simulink model "eCS_Algo_Simulation_2015b_opti"  (R2015b)
settings: Solver=ode1  StartTime=0.0  StopTime=3  FixedStep=1/80000  RelTol=1e-3
PreLoadFcn:
  | if exist('tl_preloadfcn','file'), tl_preloadfcn(gcs,402); end
PostLoadFcn:
  | , if any(exist('dsrtsu_mdlpostloadfcn', 'file') == [2, 3, 6]), try dsrtsu_mdlpostloadfcn('Execute', bdroot); catch fprintf('Error in PostLoadFcn (dsrtsu_mdlpostloadfcn) for model "%s":\n %s\n', bdroot, lasterr); end, end,
  | if exist('tl_postloadfcn','file'), tl_postloadfcn(gcs,402); end
InitFcn:
  | Omegan=1.3024e+03;
  | xi=0.9; %0.48
  | K=0.1931;
  | K1=0.0198;
  | TauLocked=0.00255;
  | TauUnLocked=0.0042;
  | Kp=1/(2*K1);
  | Ki=Kp/((TauLocked+TauUnLocked)/2);
  | if exist('tlds_init','file'), tlds_init(gcs); end
StartFcn:
  | if exist('tlds_start','file'), tlds_start(gcs); end
StopFcn:
  | if exist('tlds_stop','file'), tlds_stop(gcs); end
model workspace (MAT data in the model file):
  au8PrevExecProfile = [0 0 0 0 0 0]
values from neighbouring files (symbols this model uses):
  AccSensor = 5    [Parameter_eCS_Algo.m]
  AlgoType = 0    [Parameter_eCS_Algo.m]
  Cxy = 1*0.017    (= 0.017)    [Acc_Init_SelV1.m]
  Cxz = 1*0.017    (= 0.017)    [Acc_Init_SelV1.m]
  Cyx = 1*0.017    (= 0.017)    [Acc_Init_SelV1.m]
  Cyz = 1*0.017    (= 0.017)    [Acc_Init_SelV1.m]
  Czx = 1*0.017    (= 0.017)    [Acc_Init_SelV1.m]
  Czy = 1*0.017    (= 0.017)    [Acc_Init_SelV1.m]
  Forced_Oscillation = 0    [Parameter_eCS_Algo.m]    (also in run_Rotation_sim.m = run)
  FreqTemperature = 10    [Acc_Init_SelV1.m]
  MaxSensorOffset = 0.3    [Acc_Init_SelV1.m]
  Mean_x_noise = 4e-3    (= 0.004)    [Acc_Init_SelV1.m]
  Mean_y_noise = 4e-3    (= 0.004)    [Acc_Init_SelV1.m]
  Mean_z_noise = 4e-3    (= 0.004)    [Acc_Init_SelV1.m]
  ODR = 8000    [Acc_Init_SelV1.m]
  offsetcorrection_on_off = 0    [Parameter_eCS_Algo.m]
  phi_pulse_rotation = 0    [Parameter_eCS_Algo.m]    (also in run_Rotation_sim.m = angle)
  pulsetype = 2    [Parameter_eCS_Algo.m]    (also in run_simulation.m = j; run_simulation_ActiveX.m = j)
  Range = 4    [Acc_Init_SelV1.m]
  sensitivity_optimisation = 0    [Parameter_eCS_Algo.m]
  TempBias = 0    [Acc_Init_SelV1.m]
  TemperatureAmp = 0    [Acc_Init_SelV1.m]
  Var_x_noise = 1.84e-9    (= 1.84e-09)    [Acc_Init_SelV1.m]
  Var_y_noise = 2.025e-09    [Acc_Init_SelV1.m]
  Var_z_noise = 1.374e-09    [Acc_Init_SelV1.m]
  w_x = 2*pi*F_x    (= 376.991118431)    [Acc_Init_SelV1.m]
  w_y = 2*pi*F_y    (= 376.991118431)    [Acc_Init_SelV1.m]
  w_z = 2*pi*F_z    (= 376.991118431)    [Acc_Init_SelV1.m]
  x_max_temp_drift = 0.061    [Acc_Init_SelV1.m]
  x_offset_enable = 0    [Acc_Init_SelV1.m]
  x_run_to_run_drift = 0.0    (= 0)    [Acc_Init_SelV1.m]
  x_temp_co_drift = 0.000    (= 0)    [Acc_Init_SelV1.m]
  Xi_x = 0.7    [Acc_Init_SelV1.m]
  Xi_y = 0.7    [Acc_Init_SelV1.m]
  Xi_z = 0.7    [Acc_Init_SelV1.m]
  y_max_temp_drift = 0.061    [Acc_Init_SelV1.m]
  y_offset_enable = 0    [Acc_Init_SelV1.m]
  y_run_to_run_drift = 0.0    (= 0)    [Acc_Init_SelV1.m]
  y_temp_co_drift = 0.000    (= 0)    [Acc_Init_SelV1.m]
  z_max_temp_drift = 0.13    [Acc_Init_SelV1.m]
  z_offset_enable = 0    [Acc_Init_SelV1.m]
  z_run_to_run_drift = 0.0    (= 0)    [Acc_Init_SelV1.m]
  z_temp_co_drift = 0.000    (= 0)    [Acc_Init_SelV1.m]
undefined symbols (not defined in the file or in its folder): ddv, DiscIntNeverNeededParam, gmw_roada_x__m_s__, gmw_roada_y__m_s__, gmw_roadtime_2kHz, KSF_50_a_x, KSF_50_a_y, KSF_50_time, KSG_30_a_x, KSG_30_a_y, KSG_30_time, Meldorf_HindenburgstraAcceleration_x__m_s_2_, Meldorf_HindenburgstraAcceleration_y__m_s_2_, Meldorf_HindenburgstraAcceleration_z__m_s_2_, Meldorf_HindenburgstraTime__s_, pulse_FF27, pulse_MPDB, pulse_ODB40, pulse_ODB64, pulse_USNCAP, pulsetime_FF27, pulsetime_MPDB, pulsetime_ODB40, pulsetime_ODB64, pulsetime_USNCAP, Rauasphalt_60_a_x, Rauasphalt_60_a_y, Rauasphalt_60_time, sigbuilder_block, VW_416_2kHza_x_2kHz, VW_416_2kHza_y_2kHz, VW_416_2kHztime_2kHz
libraries: simulink x20, tllib x14, tl_autosar_lib x9, simulink_extras x7, LIB_TF_G_12_StepControl x2, LIB_TF_G_111 x1, LIB_TF_G_112 x1
(part 5 of 8)

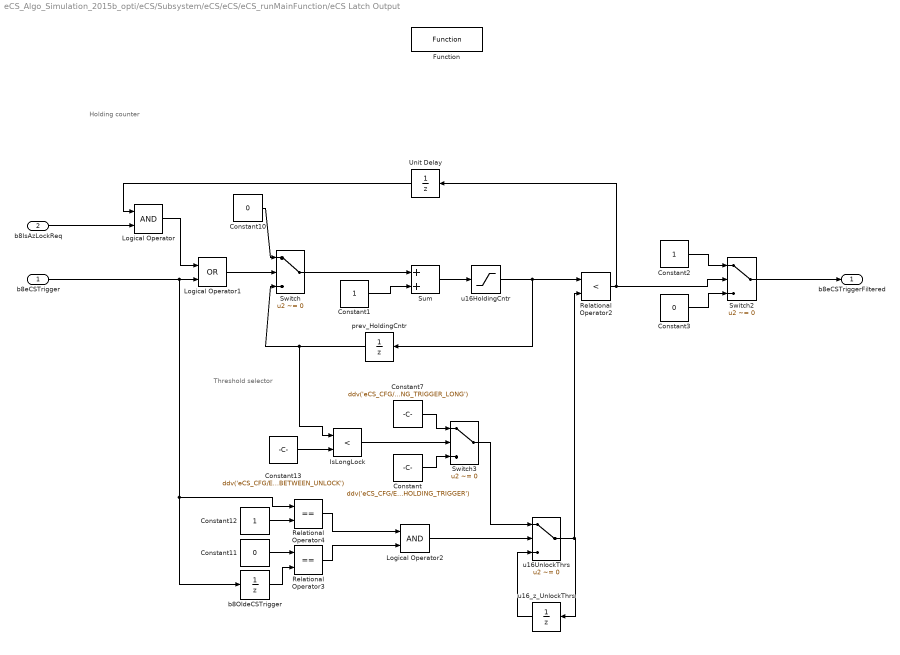
== system eCS_Algo_Simulation_2015b_opti/eCS/Subsystem/eCS/eCS/eCS_runMainFunction/eCS Latch Output ==
  note: Threshold selector
  note: Holding counter
  b8eCSTrigger : Inport
  b8IsAzLockReq : Inport  Port=2
  Constant : Constant  Value=ddv('eCS_CFG/ECS_HOLDING_TRIGGER')  mask(TL_Constant){data={'output',{'variable','eCS_CFG/ECS_HOLDING_TRIGGER'},'date',738573.71920614585}}
      settings: CopyFcn=if exist('tl_reset_reviewflag') == 2, tl_reset_reviewflag(gcbh); end  DeleteFcn=if exist('delete_tlblock','file')==2,delete_tlblock(gcbh);end  NameChangeFcn=if exist('rename_tlblock','file')==2,rename_tlblock(gcbh);end  OpenFcn=if exist('tl_open_blockdlg','file')==2,tl_open_blockdlg(gcbh);else,open_system(gcbh,'parameter');end
      mask Help: eval(['if exist(''tl_online_help'',''file'') == 2, tl_online_help(''Topic'',''TL_Constant''),else, web([''jar:file:///'',matlabroot,''/help/toolbox/simulink/help.jar!/slref/' lower(get_param(gcbh,'Blocktype')) '.html''], ''-helpbrowser''),end'])
      mask Display: plot([-0.1, 1.05, NaN, -0.1, 1.05],[.01, .01, NaN, .99, .99]);
  Constant1 : Constant  mask(TL_Constant){data={'date',738573.71920634259}}
      settings: CopyFcn=if exist('tl_reset_reviewflag') == 2, tl_reset_reviewflag(gcbh); end  DeleteFcn=if exist('delete_tlblock','file')==2,delete_tlblock(gcbh);end  NameChangeFcn=if exist('rename_tlblock','file')==2,rename_tlblock(gcbh);end  OpenFcn=if exist('tl_open_blockdlg','file')==2,tl_open_blockdlg(gcbh);else,open_system(gcbh,'parameter');end
      mask Help: eval(['if exist(''tl_online_help'',''file'') == 2, tl_online_help(''Topic'',''TL_Constant''),else, web([''jar:file:///'',matlabroot,''/help/toolbox/simulink/help.jar!/slref/' lower(get_param(gcbh,'Blocktype')) '.html''], ''-helpbrowser''),end'])
      mask Display: plot([-0.1, 1.05, NaN, -0.1, 1.05],[.01, .01, NaN, .99, .99]);
  Constant10 : Constant  Value=0  mask(TL_Constant){data={'date',738573.71920648147}}
      settings: CopyFcn=if exist('tl_reset_reviewflag') == 2, tl_reset_reviewflag(gcbh); end  DeleteFcn=if exist('delete_tlblock','file')==2,delete_tlblock(gcbh);end  NameChangeFcn=if exist('rename_tlblock','file')==2,rename_tlblock(gcbh);end  OpenFcn=if exist('tl_open_blockdlg','file')==2,tl_open_blockdlg(gcbh);else,open_system(gcbh,'parameter');end
      mask Help: eval(['if exist(''tl_online_help'',''file'') == 2, tl_online_help(''Topic'',''TL_Constant''),else, web([''jar:file:///'',matlabroot,''/help/toolbox/simulink/help.jar!/slref/' lower(get_param(gcbh,'Blocktype')) '.html''], ''-helpbrowser''),end'])
      mask Display: plot([-0.1, 1.05, NaN, -0.1, 1.05],[.01, .01, NaN, .99, .99]);
  Constant11 : Constant  Value=0  mask(TL_Constant){data={'date',738573.71920659719}}
      settings: CopyFcn=if exist('tl_reset_reviewflag') == 2, tl_reset_reviewflag(gcbh); end  DeleteFcn=if exist('delete_tlblock','file')==2,delete_tlblock(gcbh);end  NameChangeFcn=if exist('rename_tlblock','file')==2,rename_tlblock(gcbh);end  OpenFcn=if exist('tl_open_blockdlg','file')==2,tl_open_blockdlg(gcbh);else,open_system(gcbh,'parameter');end
      mask Help: eval(['if exist(''tl_online_help'',''file'') == 2, tl_online_help(''Topic'',''TL_Constant''),else, web([''jar:file:///'',matlabroot,''/help/toolbox/simulink/help.jar!/slref/' lower(get_param(gcbh,'Blocktype')) '.html''], ''-helpbrowser''),end'])
      mask Display: plot([-0.1, 1.05, NaN, -0.1, 1.05],[.01, .01, NaN, .99, .99]);
  Constant12 : Constant  mask(TL_Constant){data={'date',738573.71920671291}}
      settings: CopyFcn=if exist('tl_reset_reviewflag') == 2, tl_reset_reviewflag(gcbh); end  DeleteFcn=if exist('delete_tlblock','file')==2,delete_tlblock(gcbh);end  NameChangeFcn=if exist('rename_tlblock','file')==2,rename_tlblock(gcbh);end  OpenFcn=if exist('tl_open_blockdlg','file')==2,tl_open_blockdlg(gcbh);else,open_system(gcbh,'parameter');end
      mask Help: eval(['if exist(''tl_online_help'',''file'') == 2, tl_online_help(''Topic'',''TL_Constant''),else, web([''jar:file:///'',matlabroot,''/help/toolbox/simulink/help.jar!/slref/' lower(get_param(gcbh,'Blocktype')) '.html''], ''-helpbrowser''),end'])
      mask Display: plot([-0.1, 1.05, NaN, -0.1, 1.05],[.01, .01, NaN, .99, .99]);
  Constant13 : Constant  Value=ddv('eCS_CFG/ECS_DELAY_BETWEEN_UNLOCK')  mask(TL_Constant){data={'output',{'variable','eCS_CFG/ECS_DELAY_BETWEEN_UNLOCK'},'date',738573.71920692129}}
      settings: CopyFcn=if exist('tl_reset_reviewflag') == 2, tl_reset_reviewflag(gcbh); end  DeleteFcn=if exist('delete_tlblock','file')==2,delete_tlblock(gcbh);end  NameChangeFcn=if exist('rename_tlblock','file')==2,rename_tlblock(gcbh);end  OpenFcn=if exist('tl_open_blockdlg','file')==2,tl_open_blockdlg(gcbh);else,open_system(gcbh,'parameter');end
      mask Help: eval(['if exist(''tl_online_help'',''file'') == 2, tl_online_help(''Topic'',''TL_Constant''),else, web([''jar:file:///'',matlabroot,''/help/toolbox/simulink/help.jar!/slref/' lower(get_param(gcbh,'Blocktype')) '.html''], ''-helpbrowser''),end'])
      mask Display: plot([-0.1, 1.05, NaN, -0.1, 1.05],[.01, .01, NaN, .99, .99]);
  Constant2 : Constant  mask(TL_Constant){data={'date',738573.71920706017}}
      settings: CopyFcn=if exist('tl_reset_reviewflag') == 2, tl_reset_reviewflag(gcbh); end  DeleteFcn=if exist('delete_tlblock','file')==2,delete_tlblock(gcbh);end  NameChangeFcn=if exist('rename_tlblock','file')==2,rename_tlblock(gcbh);end  OpenFcn=if exist('tl_open_blockdlg','file')==2,tl_open_blockdlg(gcbh);else,open_system(gcbh,'parameter');end
      mask Help: eval(['if exist(''tl_online_help'',''file'') == 2, tl_online_help(''Topic'',''TL_Constant''),else, web([''jar:file:///'',matlabroot,''/help/toolbox/simulink/help.jar!/slref/' lower(get_param(gcbh,'Blocktype')) '.html''], ''-helpbrowser''),end'])
      mask Display: plot([-0.1, 1.05, NaN, -0.1, 1.05],[.01, .01, NaN, .99, .99]);
  Constant3 : Constant  Value=0  mask(TL_Constant){data={'date',738573.71920717589}}
      settings: CopyFcn=if exist('tl_reset_reviewflag') == 2, tl_reset_reviewflag(gcbh); end  DeleteFcn=if exist('delete_tlblock','file')==2,delete_tlblock(gcbh);end  NameChangeFcn=if exist('rename_tlblock','file')==2,rename_tlblock(gcbh);end  OpenFcn=if exist('tl_open_blockdlg','file')==2,tl_open_blockdlg(gcbh);else,open_system(gcbh,'parameter');end
      mask Help: eval(['if exist(''tl_online_help'',''file'') == 2, tl_online_help(''Topic'',''TL_Constant''),else, web([''jar:file:///'',matlabroot,''/help/toolbox/simulink/help.jar!/slref/' lower(get_param(gcbh,'Blocktype')) '.html''], ''-helpbrowser''),end'])
      mask Display: plot([-0.1, 1.05, NaN, -0.1, 1.05],[.01, .01, NaN, .99, .99]);
  Constant7 : Constant  Value=ddv('eCS_CFG/ECS_HOLDING_TRIGGER_LONG')  mask(TL_Constant){data={'output',{'variable','eCS_CFG/ECS_HOLDING_TRIGGER_LONG'},'date',738573.71920729172}}
      settings: CopyFcn=if exist('tl_reset_reviewflag') == 2, tl_reset_reviewflag(gcbh); end  DeleteFcn=if exist('delete_tlblock','file')==2,delete_tlblock(gcbh);end  NameChangeFcn=if exist('rename_tlblock','file')==2,rename_tlblock(gcbh);end  OpenFcn=if exist('tl_open_blockdlg','file')==2,tl_open_blockdlg(gcbh);else,open_system(gcbh,'parameter');end
      mask Help: eval(['if exist(''tl_online_help'',''file'') == 2, tl_online_help(''Topic'',''TL_Constant''),else, web([''jar:file:///'',matlabroot,''/help/toolbox/simulink/help.jar!/slref/' lower(get_param(gcbh,'Blocktype')) '.html''], ''-helpbrowser''),end'])
      mask Display: plot([-0.1, 1.05, NaN, -0.1, 1.05],[.01, .01, NaN, .99, .99]);
  Function : tllib/Function  data={'stepfunctionname','eCS_LatchTrigger','date',738077.45310667821}  displayString=FUNCTION
  IsLongLock : RelationalOperator  Operator=<  OutDataTypeStr=boolean  mask(TL_RelationalOperator){data={'date',738573.71920749999}}
      settings: DeleteFcn=if exist('delete_tlblock','file')==2,delete_tlblock(gcbh);end  NameChangeFcn=if exist('rename_tlblock','file')==2,rename_tlblock(gcbh);end  OpenFcn=if exist('tl_open_blockdlg','file')==2,tl_open_blockdlg(gcbh);else,open_system(gcbh,'parameter');end
      mask Help: eval(['if exist(''tl_online_help'',''file'') == 2, tl_online_help(''Topic'',''TL_RelationalOperator''),else, web([''jar:file:///'',matlabroot,''/help/toolbox/simulink/help.jar!/slref/' lower(get_param(gcbh,'Blocktype')) '.html''], ''-helpbrowser''),end'])
      mask Display: plot([-0.1, 1.05, NaN, -0.1, 1.05],[.01, .01, NaN, .99, .99]);
  Logical Operator : Logic  AllPortsSameDT=off  OutDataTypeStr=boolean  mask(TL_LogicalOperator){data={'date',738573.71920762735}}
      settings: DeleteFcn=if exist('delete_tlblock','file')==2,delete_tlblock(gcbh);end  NameChangeFcn=if exist('rename_tlblock','file')==2,rename_tlblock(gcbh);end  OpenFcn=if exist('tl_open_blockdlg','file')==2,tl_open_blockdlg(gcbh);else,open_system(gcbh,'parameter');end
      mask Help: eval(['if exist(''tl_online_help'',''file'') == 2, tl_online_help(''Topic'',''TL_LogicalOperator''),else, web([''jar:file:///'',matlabroot,''/help/toolbox/simulink/help.jar!/slref/' lower(get_param(gcbh,'Blocktype')) '.html''], ''-helpbrowser''),end'])
      mask Display: plot([-0.1, 1.05, NaN, -0.1, 1.05],[.01, .01, NaN, .99, .99]);
  Logical Operator1 : Logic  Operator=OR  AllPortsSameDT=off  OutDataTypeStr=boolean  mask(TL_LogicalOperator){data={'date',738573.71920774307}}
      settings: DeleteFcn=if exist('delete_tlblock','file')==2,delete_tlblock(gcbh);end  NameChangeFcn=if exist('rename_tlblock','file')==2,rename_tlblock(gcbh);end  OpenFcn=if exist('tl_open_blockdlg','file')==2,tl_open_blockdlg(gcbh);else,open_system(gcbh,'parameter');end
      mask Help: eval(['if exist(''tl_online_help'',''file'') == 2, tl_online_help(''Topic'',''TL_LogicalOperator''),else, web([''jar:file:///'',matlabroot,''/help/toolbox/simulink/help.jar!/slref/' lower(get_param(gcbh,'Blocktype')) '.html''], ''-helpbrowser''),end'])
      mask Display: plot([-0.1, 1.05, NaN, -0.1, 1.05],[.01, .01, NaN, .99, .99]);
  Logical Operator2 : Logic  AllPortsSameDT=off  OutDataTypeStr=boolean  mask(TL_LogicalOperator){data={'date',738573.71920785878}}
      settings: DeleteFcn=if exist('delete_tlblock','file')==2,delete_tlblock(gcbh);end  NameChangeFcn=if exist('rename_tlblock','file')==2,rename_tlblock(gcbh);end  OpenFcn=if exist('tl_open_blockdlg','file')==2,tl_open_blockdlg(gcbh);else,open_system(gcbh,'parameter');end
      mask Help: eval(['if exist(''tl_online_help'',''file'') == 2, tl_online_help(''Topic'',''TL_LogicalOperator''),else, web([''jar:file:///'',matlabroot,''/help/toolbox/simulink/help.jar!/slref/' lower(get_param(gcbh,'Blocktype')) '.html''], ''-helpbrowser''),end'])
      mask Display: plot([-0.1, 1.05, NaN, -0.1, 1.05],[.01, .01, NaN, .99, .99]);
  Relational Operator2 : RelationalOperator  Operator=<  OutDataTypeStr=boolean  mask(TL_RelationalOperator){data={'date',738573.71920802083}}
      settings: DeleteFcn=if exist('delete_tlblock','file')==2,delete_tlblock(gcbh);end  NameChangeFcn=if exist('rename_tlblock','file')==2,rename_tlblock(gcbh);end  OpenFcn=if exist('tl_open_blockdlg','file')==2,tl_open_blockdlg(gcbh);else,open_system(gcbh,'parameter');end
      mask Help: eval(['if exist(''tl_online_help'',''file'') == 2, tl_online_help(''Topic'',''TL_RelationalOperator''),else, web([''jar:file:///'',matlabroot,''/help/toolbox/simulink/help.jar!/slref/' lower(get_param(gcbh,'Blocktype')) '.html''], ''-helpbrowser''),end'])
      mask Display: plot([-0.1, 1.05, NaN, -0.1, 1.05],[.01, .01, NaN, .99, .99]);
  Relational Operator3 : RelationalOperator  Operator===  OutDataTypeStr=boolean  mask(TL_RelationalOperator){data={'date',738573.71920814819}}
      settings: DeleteFcn=if exist('delete_tlblock','file')==2,delete_tlblock(gcbh);end  NameChangeFcn=if exist('rename_tlblock','file')==2,rename_tlblock(gcbh);end  OpenFcn=if exist('tl_open_blockdlg','file')==2,tl_open_blockdlg(gcbh);else,open_system(gcbh,'parameter');end
      mask Help: eval(['if exist(''tl_online_help'',''file'') == 2, tl_online_help(''Topic'',''TL_RelationalOperator''),else, web([''jar:file:///'',matlabroot,''/help/toolbox/simulink/help.jar!/slref/' lower(get_param(gcbh,'Blocktype')) '.html''], ''-helpbrowser''),end'])
      mask Display: plot([-0.1, 1.05, NaN, -0.1, 1.05],[.01, .01, NaN, .99, .99]);
  Relational Operator4 : RelationalOperator  Operator===  OutDataTypeStr=boolean  mask(TL_RelationalOperator){data={'date',738573.71920833329}}
      settings: DeleteFcn=if exist('delete_tlblock','file')==2,delete_tlblock(gcbh);end  NameChangeFcn=if exist('rename_tlblock','file')==2,rename_tlblock(gcbh);end  OpenFcn=if exist('tl_open_blockdlg','file')==2,tl_open_blockdlg(gcbh);else,open_system(gcbh,'parameter');end
      mask Help: eval(['if exist(''tl_online_help'',''file'') == 2, tl_online_help(''Topic'',''TL_RelationalOperator''),else, web([''jar:file:///'',matlabroot,''/help/toolbox/simulink/help.jar!/slref/' lower(get_param(gcbh,'Blocktype')) '.html''], ''-helpbrowser''),end'])
      mask Display: plot([-0.1, 1.05, NaN, -0.1, 1.05],[.01, .01, NaN, .99, .99]);
  Sum : Sum  mask(TL_Sum){data={'output',{'type','UInt16'},'date',738573.71920846065}}
      settings: CopyFcn=if exist('tl_reset_reviewflag') == 2, tl_reset_reviewflag(gcbh); end  DeleteFcn=if exist('delete_tlblock','file')==2,delete_tlblock(gcbh);end  NameChangeFcn=if exist('rename_tlblock','file')==2,rename_tlblock(gcbh);end  OpenFcn=if exist('tl_open_blockdlg','file')==2,tl_open_blockdlg(gcbh);else,open_system(gcbh,'parameter');end
      mask Help: eval(['if exist(''tl_online_help'',''file'') == 2, tl_online_help(''Topic'',''TL_Sum''),else, web([''jar:file:///'',matlabroot,''/help/toolbox/simulink/help.jar!/slref/' lower(get_param(gcbh,'Blocktype')) '.html''], ''-helpbrowser''),end'])
      mask Display: plot([-0.1, 1.05, NaN, -0.1, 1.05],[.01, .01, NaN, .99, .99]);
  Switch : Switch  Criteria=u2 ~= 0  mask(TL_Switch){data={'output',{'type','UInt16'},'date',738573.71920854168}}
      settings: CopyFcn=if exist('tl_reset_reviewflag') == 2, tl_reset_reviewflag(gcbh); end  DeleteFcn=if exist('delete_tlblock','file')==2,delete_tlblock(gcbh);end  NameChangeFcn=if exist('rename_tlblock','file')==2,rename_tlblock(gcbh);end  OpenFcn=if exist('tl_open_blockdlg','file')==2,tl_open_blockdlg(gcbh);else,open_system(gcbh,'parameter');end
      mask Help: eval(['if exist(''tl_online_help'',''file'') == 2, tl_online_help(''Topic'',''TL_Switch''),else, web([''jar:file:///'',matlabroot,''/help/toolbox/simulink/help.jar!/slref/' lower(get_param(gcbh,'Blocktype')) '.html''], ''-helpbrowser''),end'])
      mask Display: plot([-0.1, 1.05, NaN, -0.1, 1.05],[.01, .01, NaN, .99, .99]);
  Switch2 : Switch  Criteria=u2 ~= 0  mask(TL_Switch){data={'output',{'type','Bool'},'date',738573.71920869208}}
      settings: CopyFcn=if exist('tl_reset_reviewflag') == 2, tl_reset_reviewflag(gcbh); end  DeleteFcn=if exist('delete_tlblock','file')==2,delete_tlblock(gcbh);end  NameChangeFcn=if exist('rename_tlblock','file')==2,rename_tlblock(gcbh);end  OpenFcn=if exist('tl_open_blockdlg','file')==2,tl_open_blockdlg(gcbh);else,open_system(gcbh,'parameter');end
      mask Help: eval(['if exist(''tl_online_help'',''file'') == 2, tl_online_help(''Topic'',''TL_Switch''),else, web([''jar:file:///'',matlabroot,''/help/toolbox/simulink/help.jar!/slref/' lower(get_param(gcbh,'Blocktype')) '.html''], ''-helpbrowser''),end'])
      mask Display: plot([-0.1, 1.05, NaN, -0.1, 1.05],[.01, .01, NaN, .99, .99]);
  Switch3 : Switch  Criteria=u2 ~= 0  mask(TL_Switch){data={'output',{'type','UInt16'},'date',738573.7192089468}}
      settings: CopyFcn=if exist('tl_reset_reviewflag') == 2, tl_reset_reviewflag(gcbh); end  DeleteFcn=if exist('delete_tlblock','file')==2,delete_tlblock(gcbh);end  NameChangeFcn=if exist('rename_tlblock','file')==2,rename_tlblock(gcbh);end  OpenFcn=if exist('tl_open_blockdlg','file')==2,tl_open_blockdlg(gcbh);else,open_system(gcbh,'parameter');end
      mask Help: eval(['if exist(''tl_online_help'',''file'') == 2, tl_online_help(''Topic'',''TL_Switch''),else, web([''jar:file:///'',matlabroot,''/help/toolbox/simulink/help.jar!/slref/' lower(get_param(gcbh,'Blocktype')) '.html''], ''-helpbrowser''),end'])
      mask Display: plot([-0.1, 1.05, NaN, -0.1, 1.05],[.01, .01, NaN, .99, .99]);
  Unit Delay : UnitDelay  SampleTime=-1  mask(TL_UnitDelay){data={'output',{'type','Bool'},'state',{'type','Bool'},'date',738573.71920909721}}
      settings: CopyFcn=if exist('tl_reset_reviewflag') == 2, tl_reset_reviewflag(gcbh); end  DeleteFcn=if exist('delete_tlblock','file')==2,delete_tlblock(gcbh);end  NameChangeFcn=if exist('rename_tlblock','file')==2,rename_tlblock(gcbh);end  OpenFcn=if exist('tl_open_blockdlg','file')==2,tl_open_blockdlg(gcbh);else,open_system(gcbh,'parameter');end
      mask Help: eval(['if exist(''tl_online_help'',''file'') == 2, tl_online_help(''Topic'',''TL_UnitDelay''),else, web([''jar:file:///'',matlabroot,''/help/toolbox/simulink/help.jar!/slref/' lower(get_param(gcbh,'Blocktype')) '.html''], ''-helpbrowser''),end'])
      mask Display: plot([-0.1, 1.05, NaN, -0.1, 1.05],[.01, .01, NaN, .99, .99]);
  b8OldeCSTrigger : UnitDelay  SampleTime=-1  mask(TL_UnitDelay){data={'date',738573.71920924773}}
      settings: CopyFcn=if exist('tl_reset_reviewflag') == 2, tl_reset_reviewflag(gcbh); end  DeleteFcn=if exist('delete_tlblock','file')==2,delete_tlblock(gcbh);end  NameChangeFcn=if exist('rename_tlblock','file')==2,rename_tlblock(gcbh);end  OpenFcn=if exist('tl_open_blockdlg','file')==2,tl_open_blockdlg(gcbh);else,open_system(gcbh,'parameter');end
      mask Help: eval(['if exist(''tl_online_help'',''file'') == 2, tl_online_help(''Topic'',''TL_UnitDelay''),else, web([''jar:file:///'',matlabroot,''/help/toolbox/simulink/help.jar!/slref/' lower(get_param(gcbh,'Blocktype')) '.html''], ''-helpbrowser''),end'])
      mask Display: plot([-0.1, 1.05, NaN, -0.1, 1.05],[.01, .01, NaN, .99, .99]);
  prev_HoldingCntr : UnitDelay  SampleTime=-1  mask(TL_UnitDelay){data={'output',{'type','UInt16'},'state',{'type','UInt16'},'date',738573.71920953703}}
      settings: CopyFcn=if exist('tl_reset_reviewflag') == 2, tl_reset_reviewflag(gcbh); end  DeleteFcn=if exist('delete_tlblock','file')==2,delete_tlblock(gcbh);end  NameChangeFcn=if exist('rename_tlblock','file')==2,rename_tlblock(gcbh);end  OpenFcn=if exist('tl_open_blockdlg','file')==2,tl_open_blockdlg(gcbh);else,open_system(gcbh,'parameter');end
      mask Help: eval(['if exist(''tl_online_help'',''file'') == 2, tl_online_help(''Topic'',''TL_UnitDelay''),else, web([''jar:file:///'',matlabroot,''/help/toolbox/simulink/help.jar!/slref/' lower(get_param(gcbh,'Blocktype')) '.html''], ''-helpbrowser''),end'])
      mask Display: plot([-0.1, 1.05, NaN, -0.1, 1.05],[.01, .01, NaN, .99, .99]);
  u16HoldingCntr : Saturate  UpperLimit=4000  LowerLimit=0  mask(TL_Saturate){data={'logdata',{'loggingmode',1},'output',{'type','UInt16'},'date',738573.71920969908}}
      settings: CopyFcn=if exist('tl_reset_reviewflag') == 2, tl_reset_reviewflag(gcbh); end  DeleteFcn=if exist('delete_tlblock','file')==2,delete_tlblock(gcbh);end  NameChangeFcn=if exist('rename_tlblock','file')==2,rename_tlblock(gcbh);end  OpenFcn=if exist('tl_open_blockdlg','file')==2,tl_open_blockdlg(gcbh);else,open_system(gcbh,'parameter');end
      mask Help: eval(['if exist(''tl_online_help'',''file'') == 2, tl_online_help(''Topic'',''TL_Saturate''),else, web([''jar:file:///'',matlabroot,''/help/toolbox/simulink/help.jar!/slref/' lower(get_param(gcbh,'Blocktype')) '.html''], ''-helpbrowser''),end'])
      mask Display: plot([-0.1, 1.05, NaN, -0.1, 1.05],[.01, .01, NaN, .99, .99]);
  u16UnlockThrs : Switch  Criteria=u2 ~= 0  mask(TL_Switch){data={'logdata',{'loggingmode',1},'output',{'type','UInt16'},'date',738573.71920981479}}
      settings: CopyFcn=if exist('tl_reset_reviewflag') == 2, tl_reset_reviewflag(gcbh); end  DeleteFcn=if exist('delete_tlblock','file')==2,delete_tlblock(gcbh);end  NameChangeFcn=if exist('rename_tlblock','file')==2,rename_tlblock(gcbh);end  OpenFcn=if exist('tl_open_blockdlg','file')==2,tl_open_blockdlg(gcbh);else,open_system(gcbh,'parameter');end
      mask Help: eval(['if exist(''tl_online_help'',''file'') == 2, tl_online_help(''Topic'',''TL_Switch''),else, web([''jar:file:///'',matlabroot,''/help/toolbox/simulink/help.jar!/slref/' lower(get_param(gcbh,'Blocktype')) '.html''], ''-helpbrowser''),end'])
      mask Display: plot([-0.1, 1.05, NaN, -0.1, 1.05],[.01, .01, NaN, .99, .99]);
  u16_z_UnlockThrs : UnitDelay  SampleTime=-1  mask(TL_UnitDelay){data={'output',{'type','UInt16'},'state',{'type','UInt16'},'date',738573.71921006939}}
      settings: CopyFcn=if exist('tl_reset_reviewflag') == 2, tl_reset_reviewflag(gcbh); end  DeleteFcn=if exist('delete_tlblock','file')==2,delete_tlblock(gcbh);end  NameChangeFcn=if exist('rename_tlblock','file')==2,rename_tlblock(gcbh);end  OpenFcn=if exist('tl_open_blockdlg','file')==2,tl_open_blockdlg(gcbh);else,open_system(gcbh,'parameter');end
      mask Help: eval(['if exist(''tl_online_help'',''file'') == 2, tl_online_help(''Topic'',''TL_UnitDelay''),else, web([''jar:file:///'',matlabroot,''/help/toolbox/simulink/help.jar!/slref/' lower(get_param(gcbh,'Blocktype')) '.html''], ''-helpbrowser''),end'])
      mask Display: plot([-0.1, 1.05, NaN, -0.1, 1.05],[.01, .01, NaN, .99, .99]);
  b8eCSTriggerFiltered : Outport
  wires:
  b8eCSTrigger/1 -> Relational Operator4/1, b8OldeCSTrigger/1, Logical Operator1/2
  Switch/1 -> Sum/1
  Constant1/1 -> Sum/2
  Sum/1 -> u16HoldingCntr/1
  u16HoldingCntr/1 -> Relational Operator2/1, prev_HoldingCntr/1
  prev_HoldingCntr/1 -> IsLongLock/1, Switch/3
  Constant7/1 -> Switch3/1
  Constant/1 -> Switch3/3
  Switch2/1 -> b8eCSTriggerFiltered/1
  Constant10/1 -> Switch/1
  Relational Operator4/1 -> Logical Operator2/1
  Relational Operator3/1 -> Logical Operator2/2
  Constant11/1 -> Relational Operator3/1
  b8OldeCSTrigger/1 -> Relational Operator3/2
  Constant12/1 -> Relational Operator4/2
  Logical Operator2/1 -> u16UnlockThrs/2
  Switch3/1 -> u16UnlockThrs/1
  Constant13/1 -> IsLongLock/2
  IsLongLock/1 -> Switch3/2
  u16UnlockThrs/1 -> Relational Operator2/2, u16_z_UnlockThrs/1
  u16_z_UnlockThrs/1 -> u16UnlockThrs/3
  Relational Operator2/1 -> Unit Delay/1, Switch2/2
  Constant2/1 -> Switch2/1
  Constant3/1 -> Switch2/3
  b8IsAzLockReq/1 -> Logical Operator/2
  Logical Operator1/1 -> Switch/2
  Logical Operator/1 -> Logical Operator1/1
  Unit Delay/1 -> Logical Operator/1

== system eCS_Algo_Simulation_2015b_opti/FSM/Subsystem/FSM/FSM/FSM_runCheckVehicleInputs/For Iterator Subsystem/FSM_runCheckModeStatus  ==
  u32ModesToCheck : Inport  PortDimensions=1  mask(TL_Inport){data={'output',{'variable','LOCAL_FSM/u32ModesToCheck'},'date',738799.46899457171}}
      settings: CopyFcn=if exist('tl_reset_reviewflag','file')==2,tl_reset_reviewflag(gcbh);end  DeleteFcn=if exist('delete_tlblock','file')==2,delete_tlblock(gcbh);end  NameChangeFcn=if exist('rename_tlblock','file')==2,rename_tlblock(gcbh);end  OpenFcn=if exist('tl_open_blockdlg','file')==2,tl_open_blockdlg(gcbh);else,open_system(gcbh,'parameter');end
      mask Help: eval(['if exist(''tl_online_help'',''file'') == 2, tl_online_help(''Topic'',''TL_Inport''),else, web([''jar:file:///'',matlabroot,''/help/toolbox/simulink/help.jar!/slref/' lower(get_param(gcbh,'Blocktype')) '.html''], ''-helpbrowser''),end'])
      mask Display: plot([0.2 0.35 NaN 0.65 0.8],[0 1 NaN 0 1]);
  Constant : Constant  Value=ddv('Common/B_TRUE')  mask(TL_Constant){data={'output',{'variable','Common/B_TRUE'},'date',738790.47864616895}}
      settings: CopyFcn=if exist('tl_reset_reviewflag','file')==2,tl_reset_reviewflag(gcbh);end  DeleteFcn=if exist('delete_tlblock','file')==2,delete_tlblock(gcbh);end  NameChangeFcn=if exist('rename_tlblock','file')==2,rename_tlblock(gcbh);end  OpenFcn=if exist('tl_open_blockdlg','file')==2,tl_open_blockdlg(gcbh);else,open_system(gcbh,'parameter');end
      mask Help: eval(['if exist(''tl_online_help'',''file'') == 2, tl_online_help(''Topic'',''TL_Constant''),else, web([''jar:file:///'',matlabroot,''/help/toolbox/simulink/help.jar!/slref/' lower(get_param(gcbh,'Blocktype')) '.html''], ''-helpbrowser''),end'])
      mask Display: plot([-0.1, 1.05, NaN, -0.1, 1.05],[.01, .01, NaN, .99, .99]);
  Function : tllib/Function  data={'stepfunctionname','FSM_runCheckModeStatus','stepfunctionclass','EXTERN_FCN','initfunctionname','INIT_FSM_runCheckModeStatus','functionarglist',{'u32ModesToCheck';'FSM_b8_ModeStatusResult'},'autosar',{'softwarecomponent','AUTOLIV/SoftwareComponents/FSM/FSM','runnable','FSM_runCheckModeStatus'},'date',738800.40523146989}  displayString=FUNCTION
  Terminator : Terminator
  FSM_b8_ModeStatusResult : Outport  PortDimensions=1  mask(TL_Outport){data={'output',{'variable','LOCAL_FSM/FSM_b8_ModeStatusResult'},'date',738798.55828084494}}
      settings: CopyFcn=if exist('tl_reset_reviewflag','file')==2,tl_reset_reviewflag(gcbh);end  DeleteFcn=if exist('delete_tlblock','file')==2,delete_tlblock(gcbh);end  NameChangeFcn=if exist('rename_tlblock','file')==2,rename_tlblock(gcbh);end  OpenFcn=if exist('tl_open_blockdlg','file')==2,tl_open_blockdlg(gcbh);else,open_system(gcbh,'parameter');end
      mask Help: eval(['if exist(''tl_online_help'',''file'') == 2, tl_online_help(''Topic'',''TL_Outport''),else, web([''jar:file:///'',matlabroot,''/help/toolbox/simulink/help.jar!/slref/' lower(get_param(gcbh,'Blocktype')) '.html''], ''-helpbrowser''),end'])
      mask Display: plot([0.2 0.35 NaN 0.65 0.8],[0 1 NaN 0 1]);
  wires:
  Constant/1 -> FSM_b8_ModeStatusResult/1
  u32ModesToCheck/1 -> Terminator/1

== system eCS_Algo_Simulation_2015b_opti/FSM/Subsystem/FSM/FSM/FSM_runMainFunction/ExecuteState/State Default ==
  Action Port : ActionPort  ActionType=default
  Constant1 : Constant  Value=ddv('FSM/Macros/KU8_PROFILE_NONE')  mask(TL_Constant){data={'output',{'variable','FSM/Macros/KU8_PROFILE_NONE'},'date',738801.47681858798}}
      settings: CopyFcn=if exist('tl_reset_reviewflag') == 2, tl_reset_reviewflag(gcbh); end  DeleteFcn=if exist('delete_tlblock','file')==2,delete_tlblock(gcbh);end  NameChangeFcn=if exist('rename_tlblock','file')==2,rename_tlblock(gcbh);end  OpenFcn=if exist('tl_open_blockdlg','file')==2,tl_open_blockdlg(gcbh);else,open_system(gcbh,'parameter');end
      mask Help: eval(['if exist(''tl_online_help'',''file'') == 2, tl_online_help(''Topic'',''TL_Constant''),else, web([''jar:file:///'',matlabroot,''/help/toolbox/simulink/help.jar!/slref/' lower(get_param(gcbh,'Blocktype')) '.html''], ''-helpbrowser''),end'])
      mask Display: plot([-0.1, 1.05, NaN, -0.1, 1.05],[.01, .01, NaN, .99, .99]);
  u8Profile : Outport
  wires:
  Constant1/1 -> u8Profile/1

== system eCS_Algo_Simulation_2015b_opti/FSM/Subsystem/FSM/FSM/FSM_runMainFunction/ExecuteState/State Disabled ==
  Action Port : ActionPort  ActionType=case
  Constant1 : Constant  Value=ddv('FSM/Macros/KU8_PROFILE_NONE')  mask(TL_Constant){data={'output',{'variable','FSM/Macros/KU8_PROFILE_NONE'},'date',738801.4768190278}}
      settings: CopyFcn=if exist('tl_reset_reviewflag') == 2, tl_reset_reviewflag(gcbh); end  DeleteFcn=if exist('delete_tlblock','file')==2,delete_tlblock(gcbh);end  NameChangeFcn=if exist('rename_tlblock','file')==2,rename_tlblock(gcbh);end  OpenFcn=if exist('tl_open_blockdlg','file')==2,tl_open_blockdlg(gcbh);else,open_system(gcbh,'parameter');end
      mask Help: eval(['if exist(''tl_online_help'',''file'') == 2, tl_online_help(''Topic'',''TL_Constant''),else, web([''jar:file:///'',matlabroot,''/help/toolbox/simulink/help.jar!/slref/' lower(get_param(gcbh,'Blocktype')) '.html''], ''-helpbrowser''),end'])
      mask Display: plot([-0.1, 1.05, NaN, -0.1, 1.05],[.01, .01, NaN, .99, .99]);
  u8Profile : Outport
  wires:
  Constant1/1 -> u8Profile/1

== system eCS_Algo_Simulation_2015b_opti/FSM/Subsystem/FSM/FSM/FSM_runMainFunction/ExecuteState/State Lock  ==
  Action Port : ActionPort  ActionType=case
  Constant1 : Constant  Value=ddv('FSM/Macros/KU8_PROFILE_NONE')  mask(TL_Constant){data={'output',{'variable','FSM/Macros/KU8_PROFILE_NONE'},'date',738801.47681938659}}
      settings: CopyFcn=if exist('tl_reset_reviewflag') == 2, tl_reset_reviewflag(gcbh); end  DeleteFcn=if exist('delete_tlblock','file')==2,delete_tlblock(gcbh);end  NameChangeFcn=if exist('rename_tlblock','file')==2,rename_tlblock(gcbh);end  OpenFcn=if exist('tl_open_blockdlg','file')==2,tl_open_blockdlg(gcbh);else,open_system(gcbh,'parameter');end
      mask Help: eval(['if exist(''tl_online_help'',''file'') == 2, tl_online_help(''Topic'',''TL_Constant''),else, web([''jar:file:///'',matlabroot,''/help/toolbox/simulink/help.jar!/slref/' lower(get_param(gcbh,'Blocktype')) '.html''], ''-helpbrowser''),end'])
      mask Display: plot([-0.1, 1.05, NaN, -0.1, 1.05],[.01, .01, NaN, .99, .99]);
  u8Profile : Outport
  wires:
  Constant1/1 -> u8Profile/1

== system eCS_Algo_Simulation_2015b_opti/FSM/Subsystem/FSM/FSM/FSM_runMainFunction/ExecuteState/State Unlock ==
  Action Port : ActionPort  ActionType=case
  Constant2 : Constant  Value=ddv('FSM/Macros/KU8_PROFILE_UNLOCK')  mask(TL_Constant){data={'output',{'variable','FSM/Macros/KU8_PROFILE_UNLOCK'},'date',738801.47670811345}}
      settings: CopyFcn=if exist('tl_reset_reviewflag') == 2, tl_reset_reviewflag(gcbh); end  DeleteFcn=if exist('delete_tlblock','file')==2,delete_tlblock(gcbh);end  NameChangeFcn=if exist('rename_tlblock','file')==2,rename_tlblock(gcbh);end  OpenFcn=if exist('tl_open_blockdlg','file')==2,tl_open_blockdlg(gcbh);else,open_system(gcbh,'parameter');end
      mask Help: eval(['if exist(''tl_online_help'',''file'') == 2, tl_online_help(''Topic'',''TL_Constant''),else, web([''jar:file:///'',matlabroot,''/help/toolbox/simulink/help.jar!/slref/' lower(get_param(gcbh,'Blocktype')) '.html''], ''-helpbrowser''),end'])
      mask Display: plot([-0.1, 1.05, NaN, -0.1, 1.05],[.01, .01, NaN, .99, .99]);
  u8Profile : Outport
  wires:
  Constant2/1 -> u8Profile/1

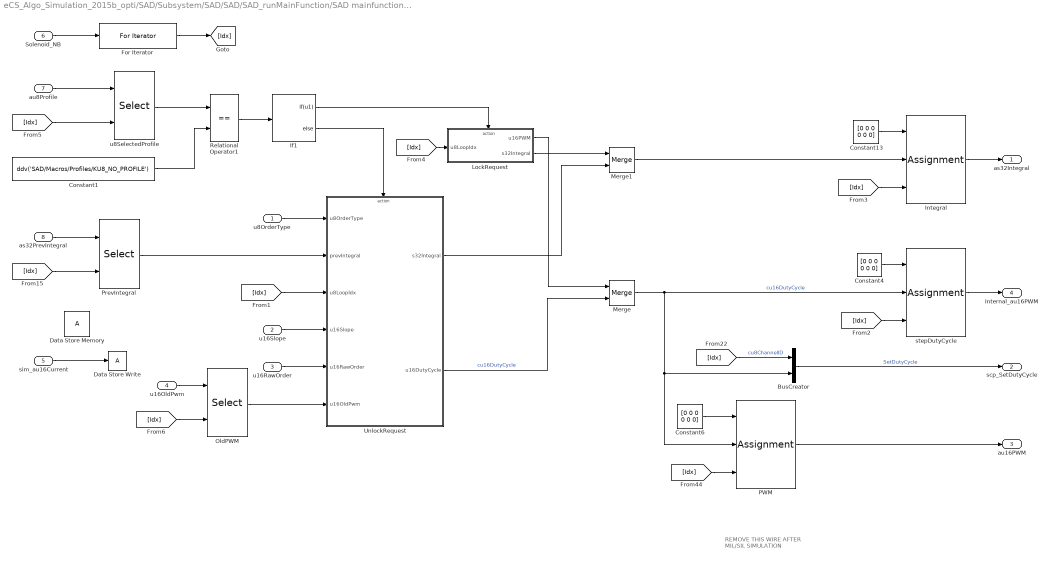
== system eCS_Algo_Simulation_2015b_opti/SAD/Subsystem/SAD/SAD/SAD_runMainFunction/SAD mainfunction/ComputeDutyCycle ==
  note: REMOVE THIS WIRE AFTER
      | MIL/SIL SIMULATION
  u8OrderType : Inport
  u16Slope : Inport  Port=2
  u16RawOrder : Inport  Port=3
  u16OldPwm : Inport  Port=4
  sim_au16Current : Inport  Port=5
  Solenoid_NB : Inport  Port=6
  au8Profile : Inport  Port=7
  as32PrevIntegral : Inport  Port=8
  BusCreator : BusCreator  Inputs=2
  Constant1 : Constant  Value=ddv('SAD/Macros/Profiles/KU8_NO_PROFILE')  mask(TL_Constant){data={'output',{'variable','SAD/Macros/Profiles/KU8_NO_PROFILE'},'date',738653.68494866893}}
      settings: CopyFcn=if exist('tl_reset_reviewflag') == 2, tl_reset_reviewflag(gcbh); end  DeleteFcn=if exist('delete_tlblock','file')==2,delete_tlblock(gcbh);end  NameChangeFcn=if exist('rename_tlblock','file')==2,rename_tlblock(gcbh);end  OpenFcn=if exist('tl_open_blockdlg','file')==2,tl_open_blockdlg(gcbh);else,open_system(gcbh,'parameter');end
      mask Help: eval(['if exist(''tl_online_help'',''file'') == 2, tl_online_help(''Topic'',''TL_Constant''),else, web([''jar:file:///'',matlabroot,''/help/toolbox/simulink/help.jar!/slref/' lower(get_param(gcbh,'Blocktype')) '.html''], ''-helpbrowser''),end'])
      mask Display: plot([-0.1, 1.05, NaN, -0.1, 1.05],[.01, .01, NaN, .99, .99]);
  Constant13 : Constant  Value=[0 0 0 0 0 0]  mask(TL_Constant){data={'date',738430.41691166663}}
      settings: CopyFcn=if exist('tl_reset_reviewflag') == 2, tl_reset_reviewflag(gcbh); end  DeleteFcn=if exist('delete_tlblock','file')==2,delete_tlblock(gcbh);end  NameChangeFcn=if exist('rename_tlblock','file')==2,rename_tlblock(gcbh);end  OpenFcn=if exist('tl_open_blockdlg','file')==2,tl_open_blockdlg(gcbh);else,open_system(gcbh,'parameter');end
      mask Help: eval(['if exist(''tl_online_help'',''file'') == 2, tl_online_help(''Topic'',''TL_Constant''),else, web([''jar:file:///'',matlabroot,''/help/toolbox/simulink/help.jar!/slref/' lower(get_param(gcbh,'Blocktype')) '.html''], ''-helpbrowser''),end'])
      mask Display: plot([-0.1, 1.05, NaN, -0.1, 1.05],[.01, .01, NaN, .99, .99]);
  Constant4 : Constant  Value=[0 0 0 0 0 0]  mask(TL_Constant){data={'date',738430.41691131948}}
      settings: CopyFcn=if exist('tl_reset_reviewflag') == 2, tl_reset_reviewflag(gcbh); end  DeleteFcn=if exist('delete_tlblock','file')==2,delete_tlblock(gcbh);end  NameChangeFcn=if exist('rename_tlblock','file')==2,rename_tlblock(gcbh);end  OpenFcn=if exist('tl_open_blockdlg','file')==2,tl_open_blockdlg(gcbh);else,open_system(gcbh,'parameter');end
      mask Help: eval(['if exist(''tl_online_help'',''file'') == 2, tl_online_help(''Topic'',''TL_Constant''),else, web([''jar:file:///'',matlabroot,''/help/toolbox/simulink/help.jar!/slref/' lower(get_param(gcbh,'Blocktype')) '.html''], ''-helpbrowser''),end'])
      mask Display: plot([-0.1, 1.05, NaN, -0.1, 1.05],[.01, .01, NaN, .99, .99]);
  Constant6 : Constant  Value=[0 0 0 0 0 0]  mask(TL_Constant){data={'date',738430.41691166663}}
      settings: CopyFcn=if exist('tl_reset_reviewflag') == 2, tl_reset_reviewflag(gcbh); end  DeleteFcn=if exist('delete_tlblock','file')==2,delete_tlblock(gcbh);end  NameChangeFcn=if exist('rename_tlblock','file')==2,rename_tlblock(gcbh);end  OpenFcn=if exist('tl_open_blockdlg','file')==2,tl_open_blockdlg(gcbh);else,open_system(gcbh,'parameter');end
      mask Help: eval(['if exist(''tl_online_help'',''file'') == 2, tl_online_help(''Topic'',''TL_Constant''),else, web([''jar:file:///'',matlabroot,''/help/toolbox/simulink/help.jar!/slref/' lower(get_param(gcbh,'Blocktype')) '.html''], ''-helpbrowser''),end'])
      mask Display: plot([-0.1, 1.05, NaN, -0.1, 1.05],[.01, .01, NaN, .99, .99]);
  Data Store Memory : DataStoreMemory  ReadBeforeWriteMsg=warning  WriteAfterWriteMsg=warning  WriteAfterReadMsg=warning  InitialValue=[0 0 0 0 0 0]  mask(TL_DataStoreMemory){data={'output',{'type','UInt16'},'date',738433.70621954859}}
      settings: CopyFcn=if exist('tl_reset_reviewflag') == 2, tl_reset_reviewflag(gcbh); end  DeleteFcn=if exist('delete_tlblock','file')==2,delete_tlblock(gcbh);end  NameChangeFcn=if exist('rename_tlblock','file')==2,rename_tlblock(gcbh);end  OpenFcn=if exist('tl_open_blockdlg','file')==2,tl_open_blockdlg(gcbh);else,open_system(gcbh,'parameter');end
      mask Help: eval(['if exist(''tl_online_help'',''file'') == 2, tl_online_help(''Topic'',''TL_DataStoreMemory''),else, web([''jar:file:///'',matlabroot,''/help/toolbox/simulink/help.jar!/slref/' lower(get_param(gcbh,'Blocktype')) '.html''], ''-helpbrowser''),end'])
      mask Display:
      | plot([-0.1, 1.05, NaN, -0.1, 1.05],[.01, .01, NaN, .99, .99]);
      | plot([-0.1, 1.05, NaN, -0.1, 1.05],[.01, .01, NaN, .99, .99]);
  Data Store Write : DataStoreWrite  mask(TL_DataStoreWrite){data={'date',738433.42894126161}}
      settings: DeleteFcn=if exist('delete_tlblock','file')==2,delete_tlblock(gcbh);end  NameChangeFcn=if exist('rename_tlblock','file')==2,rename_tlblock(gcbh);end  OpenFcn=if exist('tl_open_blockdlg','file')==2,tl_open_blockdlg(gcbh);else,open_system(gcbh,'parameter');end
      mask Help: eval(['if exist(''tl_online_help'',''file'') == 2, tl_online_help(''Topic'',''TL_DataStoreWrite''),else, web([''jar:file:///'',matlabroot,''/help/toolbox/simulink/help.jar!/slref/' lower(get_param(gcbh,'Blocktype')) '.html''], ''-helpbrowser''),end'])
      mask Display: plot([-0.1, 1.05, NaN, -0.1, 1.05],[.01, .01, NaN, .99, .99]);
  For Iterator : ForIterator  IterationSource=external  IterationLimit=6  IndexMode=Zero-based  IterationVariableDataType=int8
  If1 : If  IfExpression=u1
  Integral : Assignment  IndexMode=Zero-based  IndexOptions=Index vector (port)  Indices=1  OutputSizes=1  mask(TL_Assignment){data={'insideiteratedsystem',logical(1),'omitinitializations',1,'output',{'variable','SAD/Vars/Steps/as32Integral','inheritscaling',0},'date',738430.55898019671}}
      settings: CopyFcn=if exist('tl_reset_reviewflag') == 2, tl_reset_reviewflag(gcbh); end  DeleteFcn=if exist('delete_tlblock','file')==2,delete_tlblock(gcbh);end  NameChangeFcn=if exist('rename_tlblock','file')==2,rename_tlblock(gcbh);end  OpenFcn=if exist('tl_open_blockdlg','file')==2,tl_open_blockdlg(gcbh);else,open_system(gcbh,'parameter');end
      mask Help: eval(['if exist(''tl_online_help'',''file'') == 2, tl_online_help(''Topic'',''TL_Assignment''),else, web([''jar:file:///'',matlabroot,''/help/toolbox/simulink/help.jar!/slref/' lower(get_param(gcbh,'Blocktype')) '.html''], ''-helpbrowser''),end'])
      mask Display: plot([-0.1, 1.05, NaN, -0.1, 1.05],[.01, .01, NaN, .99, .99]);
  LockRequest : Subsystem  TreatAsAtomicUnit=on
  Merge : Merge  mask(TL_Merge){data={'date',738654.58814178244}}
      settings: CopyFcn=if exist('tl_reset_reviewflag') == 2, tl_reset_reviewflag(gcbh); end  DeleteFcn=if exist('delete_tlblock','file')==2,delete_tlblock(gcbh);end  NameChangeFcn=if exist('rename_tlblock','file')==2,rename_tlblock(gcbh);end  OpenFcn=if exist('tl_open_blockdlg','file')==2,tl_open_blockdlg(gcbh);else,open_system(gcbh,'parameter');end
      mask Help: eval(['if exist(''tl_online_help'',''file'') == 2, tl_online_help(''Topic'',''TL_Merge''),else, web([''jar:file:///'',matlabroot,''/help/toolbox/simulink/help.jar!/slref/' lower(get_param(gcbh,'Blocktype')) '.html''], ''-helpbrowser''),end'])
      mask Display: plot([-0.1, 1.05, NaN, -0.1, 1.05],[.01, .01, NaN, .99, .99]);
  Merge1 : Merge  mask(TL_Merge){data={'date',738654.58814178244}}
      settings: CopyFcn=if exist('tl_reset_reviewflag') == 2, tl_reset_reviewflag(gcbh); end  DeleteFcn=if exist('delete_tlblock','file')==2,delete_tlblock(gcbh);end  NameChangeFcn=if exist('rename_tlblock','file')==2,rename_tlblock(gcbh);end  OpenFcn=if exist('tl_open_blockdlg','file')==2,tl_open_blockdlg(gcbh);else,open_system(gcbh,'parameter');end
      mask Help: eval(['if exist(''tl_online_help'',''file'') == 2, tl_online_help(''Topic'',''TL_Merge''),else, web([''jar:file:///'',matlabroot,''/help/toolbox/simulink/help.jar!/slref/' lower(get_param(gcbh,'Blocktype')) '.html''], ''-helpbrowser''),end'])
      mask Display: plot([-0.1, 1.05, NaN, -0.1, 1.05],[.01, .01, NaN, .99, .99]);
  OldPWM : Selector  IndexMode=Zero-based  IndexOptions=Index vector (port)  Indices=[1 3]  OutputSizes=1
  PWM : Assignment  IndexMode=Zero-based  IndexOptions=Index vector (port)  Indices=1  OutputSizes=1  mask(TL_Assignment){data={'insideiteratedsystem',logical(1),'omitinitializations',1,'output',{'description',['Resolution:  2^-15'],'name','$D','max',[32768 32767 32767 32767 32767 32767],'min',[0 -32768 -32768 -32768 -32768 -32768],'type','UInt16','scaling','VOID_SCALING','inheritscaling',0},'date',738496.36831776623}}
      settings: CopyFcn=if exist('tl_reset_reviewflag') == 2, tl_reset_reviewflag(gcbh); end  DeleteFcn=if exist('delete_tlblock','file')==2,delete_tlblock(gcbh);end  NameChangeFcn=if exist('rename_tlblock','file')==2,rename_tlblock(gcbh);end  OpenFcn=if exist('tl_open_blockdlg','file')==2,tl_open_blockdlg(gcbh);else,open_system(gcbh,'parameter');end
      mask Help: eval(['if exist(''tl_online_help'',''file'') == 2, tl_online_help(''Topic'',''TL_Assignment''),else, web([''jar:file:///'',matlabroot,''/help/toolbox/simulink/help.jar!/slref/' lower(get_param(gcbh,'Blocktype')) '.html''], ''-helpbrowser''),end'])
      mask Display: plot([-0.1, 1.05, NaN, -0.1, 1.05],[.01, .01, NaN, .99, .99]);
  PrevIntegral : Selector  IndexMode=Zero-based  IndexOptions=Index vector (port)  Indices=[1 3]  OutputSizes=1
  Relational Operator1 : RelationalOperator  Operator===  OutDataTypeStr=boolean  mask(TL_RelationalOperator){data={'date',738653.68374475697}}
      settings: DeleteFcn=if exist('delete_tlblock','file')==2,delete_tlblock(gcbh);end  NameChangeFcn=if exist('rename_tlblock','file')==2,rename_tlblock(gcbh);end  OpenFcn=if exist('tl_open_blockdlg','file')==2,tl_open_blockdlg(gcbh);else,open_system(gcbh,'parameter');end
      mask Help: eval(['if exist(''tl_online_help'',''file'') == 2, tl_online_help(''Topic'',''TL_RelationalOperator''),else, web([''jar:file:///'',matlabroot,''/help/toolbox/simulink/help.jar!/slref/' lower(get_param(gcbh,'Blocktype')) '.html''], ''-helpbrowser''),end'])
      mask Display: plot([-0.1, 1.05, NaN, -0.1, 1.05],[.01, .01, NaN, .99, .99]);
  UnlockRequest : Subsystem  TreatAsAtomicUnit=on
  stepDutyCycle : Assignment  IndexMode=Zero-based  IndexOptions=Index vector (port)  Indices=1  OutputSizes=1  mask(TL_Assignment){data={'insideiteratedsystem',logical(1),'omitinitializations',1,'output',{'variable','SAD/Vars/Steps/au16DutyCycle','inheritscaling',0},'date',738430.41691431717}}
      settings: CopyFcn=if exist('tl_reset_reviewflag') == 2, tl_reset_reviewflag(gcbh); end  DeleteFcn=if exist('delete_tlblock','file')==2,delete_tlblock(gcbh);end  NameChangeFcn=if exist('rename_tlblock','file')==2,rename_tlblock(gcbh);end  OpenFcn=if exist('tl_open_blockdlg','file')==2,tl_open_blockdlg(gcbh);else,open_system(gcbh,'parameter');end
      mask Help: eval(['if exist(''tl_online_help'',''file'') == 2, tl_online_help(''Topic'',''TL_Assignment''),else, web([''jar:file:///'',matlabroot,''/help/toolbox/simulink/help.jar!/slref/' lower(get_param(gcbh,'Blocktype')) '.html''], ''-helpbrowser''),end'])
      mask Display: plot([-0.1, 1.05, NaN, -0.1, 1.05],[.01, .01, NaN, .99, .99]);
  u8SelectedProfile : Selector  IndexMode=Zero-based  IndexOptions=Index vector (port)  Indices=[1 3]  OutputSizes=1
  as32Integral : Outport
  scp_SetDutyCycle : Outport  Port=2  mask(TL_BusOutport){data={'#autoscaling',2,'#message',2,'#output',2,'#logdata',2,'signals',{{'SetDutyCycle',{'cu8ChannelID';'cu16DutyCycle'}}},'autosar',{'useautosarcommunication',1,'kind',4,'clientserverport','pclPwmServices','operation','SetDutyCycle'},'date',738496.45470876154}}
      settings: CopyFcn=if exist('tl_reset_reviewflag') == 2, tl_reset_reviewflag(gcbh); end  DeleteFcn=if exist('delete_tlblock','file')==2,delete_tlblock(gcbh);end  NameChangeFcn=if exist('rename_tlblock','file')==2,rename_tlblock(gcbh);end  OpenFcn=if exist('tl_open_blockdlg','file')==2,tl_open_blockdlg(gcbh);else,open_system(gcbh,'parameter');end
      mask Help: eval(['if exist(''tl_online_help'',''file'') == 2, tl_online_help(''Topic'',''TL_Outport''),else, web([''jar:file:///'',matlabroot,''/help/toolbox/simulink/help.jar!/slref/' lower(get_param(gcbh,'Blocktype')) '.html''], ''-helpbrowser''),end'])
      mask Display: plot([0.2 0.35 NaN 0.65 0.8],[0 1 NaN 0 1]);
  au16PWM : Outport  Port=3
  Internal_au16PWM : Outport  Port=4
  wires:
  u16RawOrder/1 -> UnlockRequest/5(u16RawOrder)
  u16Slope/1 -> UnlockRequest/4(u16Slope)
  sim_au16Current/1 -> Data Store Write/1
  For Iterator/1 -> [Idx]
  Solenoid_NB/1 -> For Iterator/1
  Constant1/1 -> Relational Operator1/2
  Relational Operator1/1 -> If1/1
  If1/1 -> LockRequest/Action
  If1/2 -> UnlockRequest/Action
  u8OrderType/1 -> UnlockRequest/1(u8OrderType)
  Integral/1 -> as32Integral/1
  [Idx] -> Integral/3
  Constant13/1 -> Integral/1
  [Idx] -> BusCreator/1  "cu8ChannelID"
  BusCreator/1 -> scp_SetDutyCycle/1  "SetDutyCycle"
  [Idx] -> PWM/3
  Constant6/1 -> PWM/1
  PWM/1 -> au16PWM/1
  as32PrevIntegral/1 -> PrevIntegral/1
  [Idx] -> PrevIntegral/2
  PrevIntegral/1 -> UnlockRequest/2(prevIntegral)
  [Idx] -> UnlockRequest/3(u8LoopIdx)
  stepDutyCycle/1 -> Internal_au16PWM/1
  [Idx] -> stepDutyCycle/3
  Constant4/1 -> stepDutyCycle/1
  [Idx] -> LockRequest/1(u8LoopIdx)
  LockRequest/1(u16PWM) -> Merge/1
  Merge/1 -> stepDutyCycle/2, BusCreator/2, PWM/2  "cu16DutyCycle"
  UnlockRequest/2(u16DutyCycle) -> Merge/2  "cu16DutyCycle"
  [Idx] -> u8SelectedProfile/2
  au8Profile/1 -> u8SelectedProfile/1
  u8SelectedProfile/1 -> Relational Operator1/1
  OldPWM/1 -> UnlockRequest/6(u16OldPwm)
  u16OldPwm/1 -> OldPWM/1
  [Idx] -> OldPWM/2
  LockRequest/2(s32Integral) -> Merge1/1
  UnlockRequest/1(s32Integral) -> Merge1/2
  Merge1/1 -> Integral/2
